simulink model "sensors"  (R2015a)
settings: Solver=ode45  StartTime=0.0  StopTime=10.0  RelTol=1e-3
libraries: vrlib x1
settings Model: Creator=johnz  LastModifiedBy=johnz

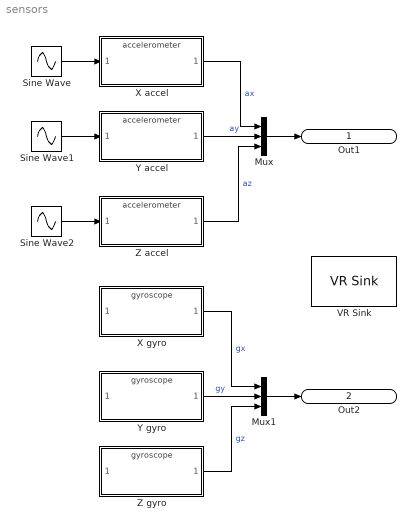
== system sensors ==
  Mux : Mux  Inputs=3
  Mux1 : Mux  Inputs=3
  Sine Wave : Sin  SampleTime=0
  Sine Wave1 : Sin  Phase=pi/4  SampleTime=0
  Sine Wave2 : Sin  Phase=pi/2  SampleTime=0
  VR Sink : vrlib/VR Sink  InstantiateOnLoad=on  SampleTime=0.1  ViewEnable=on  RemoteChange=off  RemoteView=off  WorldFileName=C:\projects\flight\math\Matlab\animation\animation_world.wrl  AutoView=off  VideoDimensions=[]  AllowVariableSize=off
  X accel : ModelReference  ModelNameDialog=accelerometer.slx  ParameterArgumentNames=randomSeed  ParameterArgumentValues=11  SimulationMode=Normal  ModelReferenceVersion=1.22  CopyOfModelName=accelerometer.slx
  X gyro : ModelReference  ModelNameDialog=gyroscope.slx  ParameterArgumentNames=randomSeed  ParameterArgumentValues=19  SimulationMode=Normal  ModelReferenceVersion=1.23  CopyOfModelName=gyroscope.slx
  Y accel : ModelReference  ModelNameDialog=accelerometer.slx  ParameterArgumentNames=randomSeed  ParameterArgumentValues=13  SimulationMode=Normal  ModelReferenceVersion=1.22  CopyOfModelName=accelerometer.slx
  Y gyro : ModelReference  ModelNameDialog=gyroscope.slx  ParameterArgumentNames=randomSeed  ParameterArgumentValues=23  SimulationMode=Normal  ModelReferenceVersion=1.23  CopyOfModelName=gyroscope.slx
  Z accel : ModelReference  ModelNameDialog=accelerometer.slx  ParameterArgumentNames=randomSeed  ParameterArgumentValues=17  SimulationMode=Normal  ModelReferenceVersion=1.22  CopyOfModelName=accelerometer.slx
  Z gyro : ModelReference  ModelNameDialog=gyroscope.slx  ParameterArgumentNames=randomSeed  ParameterArgumentValues=29  SimulationMode=Normal  ModelReferenceVersion=1.23  CopyOfModelName=gyroscope.slx
  Out1 : Outport
  Out2 : Outport  Port=2
  wires:
  X accel/1 -> Mux/1  "ax"
  Y accel/1 -> Mux/2  "ay"
  Z accel/1 -> Mux/3  "az"
  X gyro/1 -> Mux1/1  "gx"
  Y gyro/1 -> Mux1/2  "gy"
  Z gyro/1 -> Mux1/3  "gz"
  Mux/1 -> Out1/1
  Mux1/1 -> Out2/1
  Sine Wave/1 -> X accel/1
  Sine Wave1/1 -> Y accel/1
  Sine Wave2/1 -> Z accel/1
